simulink model "mcu_flat"  (R2025b)
settings: Solver=FixedStepDiscrete  StartTime=0.0  StopTime=10.0  FixedStep=Ts_inner  RelTol=1e-3
InitFcn:
  | fctrl = init_flatness(quadcop);
  | [mahony, luen] = init_estimator(fctrl.Ts_slow); % Ts_slow = 0.01 = Ts_gcs
  | xi0 = [quadcop.x0; quadcop.v0]; % Luenberger-Startzustand [p;v]
undefined symbols (not defined in the file): imu, luen, mahony, quadcop, safety, supervisor, Ts_batt, Ts_gcs, Ts_inner
settings Model: DataDictionary=project.sldd  Creator=Nick  LastModifiedBy=Rakete
settings SolverCC: AutoInsertRateTranBlk=on
settings OptimizationCC: DefaultParameterBehavior=Inlined  EnhancedBackFolding=on  PassReuseOutputArgsAs=Individual arguments  ZeroExternalMemoryAtStartup=off  ZeroInternalMemoryAtStartup=off  OptimizeBlockOrder=speed  DifferentSizesBufferReuse=on  OptimizationCustomize=off  EfficientTunableParamExpr=on
settings DebuggingCC: ParameterTunabilityLossMsg=error
settings HardwareCC: ProdBitPerPointer=32.0  ProdBitPerSizeT=32.0  ProdBitPerPtrDiffT=32.0  ProdLargestAtomicInteger=Long  ProdLargestAtomicFloat=Double  ProdWordSize=32.0  ProdLongLongMode=on  ProdHWDeviceType=ARM Compatible->ARM Cortex-M
settings SFSimCC: MATLABDynamicMemAlloc=off
settings RTWCC: SystemTargetFile=ert.tlc  GenCodeOnly=on  PackageGeneratedCodeAndArtifacts=on  TemplateMakefile=ert_default_tmf  GenerateReport=on  TargetLang=C++  Description=Embedded Coder
settings CodeAppCC: ForceParamTrailComments=on  IgnoreCustomStorageClasses=off  OperatorAnnotations=on  SimulinkDataObjDesc=on  SFDataObjDesc=on  InsertBlockDesc=on
settings ERTTargetCC: RootIOFormat=Structure reference  ERTCustomFileTemplate=example_file_process.tlc  TargetLangStandard=C++11 (ISO)  GenerateSampleERTMain=on  CodeInterfacePackaging=C++ class  SubcomponentCodeInterfacePackaging=C++ class  SupportNonFinite=off

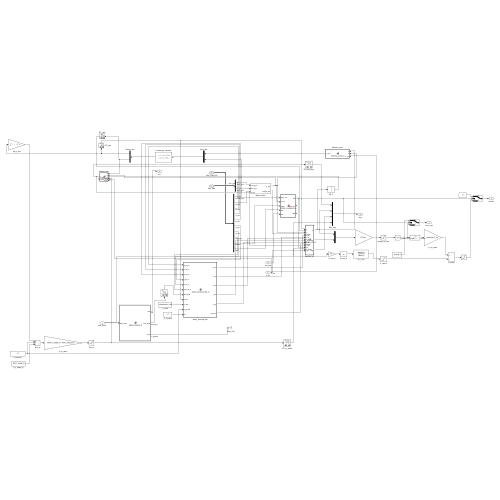
[thumbnail: Simulink's stored preview of the top-level diagram]
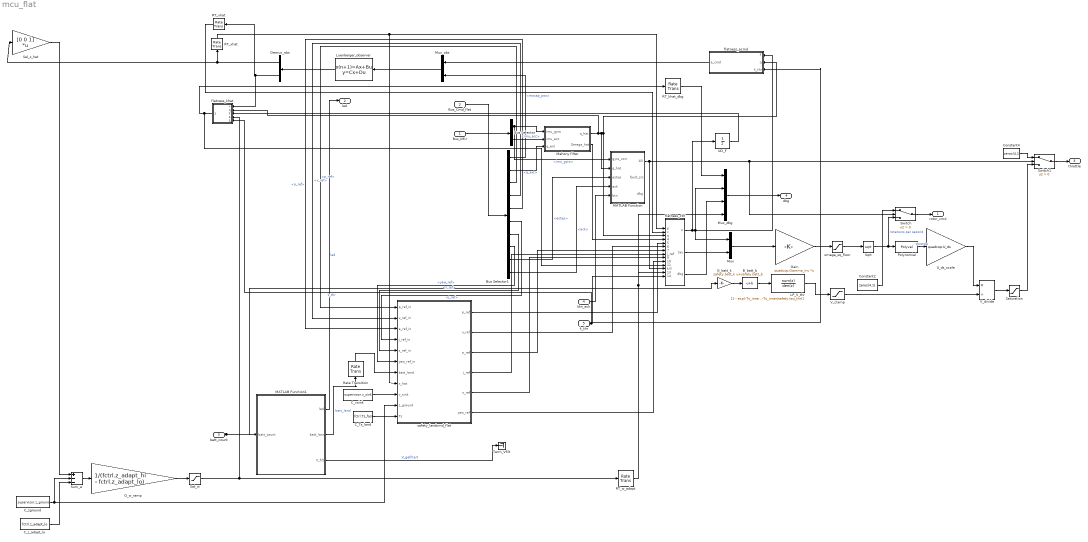
== system mcu_flat ==
  Bus_IMU : Inport  OutDataTypeStr=Bus: Bus_IMU
  Bus_Cmd_flat : Inport  Port=2  OutDataTypeStr=Bus: Bus_Cmd_flat
  batt_count : Inport  Port=3
  btn_ack : Inport  Port=4  OutDataTypeStr=boolean
  k_thr : Inport  Port=5  OutDataTypeStr=double  PortDimensions=1
  B_batt_b : Bias  Bias=safety.batt_b  SaturateOnIntegerOverflow=off
  Bus Selector : BusSelector  OutputSignals=imu_gyro,imu_acc
  Bus Selector1 : BusSelector  OutputSignals=mocap_pos,q_ext,p_ref,v_ref,a_ref,j_ref,s_ref,yaw_ref,estop,ack
  C_Ts_land : Constant  Value=fctrl.Ts_fast
  C_vsink : Constant  Value=supervisor.v_sink
  C_z_adapt_lo : Constant  Value=fctrl.z_adapt_lo
  C_zground : Constant  Value=supervisor.z_ground
  Constant2 : Constant  Value=zeros(4,1)
  Constant4 : Constant  Value=zeros(4,1)
  Demux_obs : Demux  Outputs=2
  G_batt_k : Gain  Gain=safety.batt_k
  G_w_ramp : Gain  Gain=1/(fctrl.z_adapt_hi - fctrl.z_adapt_lo)
  Gain : Gain  Gain=quadcop.Gamma_inv  Multiplication=Matrix(K*u) (u vector)
  LP_V_thr : DiscreteTransferFcn  Numerator=[1 - exp(-Ts_inner/safety.tau_thr)]  Denominator=[1, -exp(-Ts_inner/safety.tau_thr)]  InitialStates=quadcop.V_thr_init  SampleTime=Ts_inner
  Luenberger_observer : DiscreteStateSpace  A=luen.Ad  B=luen.Bd  C=luen.Cd  D=luen.Dd  InitialCondition=xi0  SampleTime=Ts_gcs
  MATLAB Function : MATLAB Function  TreatAsAtomicUnit=on
  MATLAB Function1 : MATLAB Function  TreatAsAtomicUnit=on  SystemSampleTime=Ts_batt
  Mahony filter : Subsystem
  Mux : Mux  Inputs=2
  Mux_dbg : Mux
  Mux_obs : Mux  Inputs=2
  Polynomial : Polyval  Coefs=quadcop.p_from_omega
  RT_khat_dbg : RateTransition  InitialCondition=fctrl.k_hat0
  RT_vhat : RateTransition  OutPortSampleTime=fctrl.Ts_fast
  RT_w_adapt : RateTransition
  RT_xhat : RateTransition  OutPortSampleTime=fctrl.Ts_fast
  Rate Transition : RateTransition  OutPortSampleTime=Ts_inner
  Sat_w : Saturate  UpperLimit=1  LowerLimit=0
  Saturation : Saturate  UpperLimit=100  LowerLimit=0
  Sel_z_hat : Gain  Gain=[0 0 1]  Multiplication=Matrix(K*u)
  Sqrt : Sqrt
  Sum_w : Sum  Inputs=+--
  Switch : Switch  Criteria=u2 > Threshold  SaturateOnIntegerOverflow=off  InputSameDT=off
  Switch1 : Switch  Criteria=u2 > Threshold  SaturateOnIntegerOverflow=off  InputSameDT=off
  Term_Vfilt : Terminator
  UD_F : UnitDelay  InitialCondition=fctrl.m*fctrl.g  SampleTime=fctrl.Ts_fast  HasFrameUpgradeWarning=on
  U_ds_scale : Gain  Gain=quadcop.U_ds
  V_clamp : Saturate  UpperLimit=quadcop.V_thr_max  LowerLimit=quadcop.V_thr_min
  V_divide : Product  Inputs=*/
  flatness_acmd : MATLAB Function  TreatAsAtomicUnit=on
  flatness_ctrl : MATLAB Function  TreatAsAtomicUnit=on  SystemSampleTime=fctrl.Ts_fast
  flatness_khat : MATLAB Function  TreatAsAtomicUnit=on  SystemSampleTime=fctrl.Ts_slow
  omega_sq_floor : Saturate  UpperLimit=inf  LowerLimit=0
  safety_landcmd_flat : MATLAB Function  TreatAsAtomicUnit=on  SystemSampleTime=Ts_inner
  rotor_cmd : Outport
  led : Outport  Port=2
  throttle : Outport  Port=3
  dbg : Outport  Port=4
  wires:
  Bus Selector/1 -> MATLAB Function/1(gyro_corr), Mahony filter/1(imu_gyro)  "<imu_gyro>"
  G_w_ramp/1 -> Sat_w/1
  Constant4/1 -> Switch1/1
  Sum_w/1 -> G_w_ramp/1
  C_z_adapt_lo/1 -> Sum_w/3
  Sel_z_hat/1 -> Sum_w/1
  flatness_khat/1(k_hat) -> flatness_ctrl/11(k_hat), RT_khat_dbg/1
  C_Ts_land/1 -> safety_landcmd_flat/11(Ts)
  C_zground/1 -> safety_landcmd_flat/10(z_ground), Sum_w/2
  Sat_w/1 -> flatness_khat/4(w_adapt), RT_w_adapt/1
  RT_vhat/1 -> flatness_ctrl/2(v)
  Mux_obs/1 -> Luenberger_observer/1
  RT_xhat/1 -> flatness_ctrl/1(p), safety_landcmd_flat/8(x_hat)
  batt_count/1 -> MATLAB Function1/1(batt_count), G_batt_k/1
  Demux_obs/2 -> RT_vhat/1, flatness_khat/1(v)
  Gain/1 -> omega_sq_floor/1
  Demux_obs/1 -> RT_xhat/1, Sel_z_hat/1
  MATLAB Function1/1(led) -> led/1  "led"
  C_vsink/1 -> safety_landcmd_flat/9(v_sink)
  MATLAB Function1/2(batt_land) -> Rate Transition/1  "batt_land"
  omega_sq_floor/1 -> Sqrt/1
  Mux/1 -> Gain/1
  safety_landcmd_flat/6(yaw_ref) -> flatness_ctrl/10(yawref)
  Bus Selector/2 -> Mahony filter/2(imu_acc)  "<imu_acc>"
  Luenberger_observer/1 -> Demux_obs/1
  Constant2/1 -> Switch/1
  safety_landcmd_flat/2(v_ref) -> flatness_ctrl/6(v_ref)
  Rate Transition/1 -> safety_landcmd_flat/7(batt_land)
  Bus_IMU/1 -> Bus Selector/1
  Bus_Cmd_flat/1 -> Bus Selector1/1
  Bus Selector1/5 -> safety_landcmd_flat/3(a_ref_in)  "<a_ref>"
  safety_landcmd_flat/1(p_ref) -> flatness_ctrl/5(p_ref)
  RT_khat_dbg/1 -> Mux_dbg/1
  safety_landcmd_flat/3(a_ref) -> flatness_ctrl/7(a_ref)
  U_ds_scale/1 -> V_divide/1
  Polynomial/1 -> U_ds_scale/1  "throttle"
  Sqrt/1 -> Polynomial/1, Switch/3  "rotations per second"
  Mahony filter/2(Omega_hat) -> flatness_ctrl/4(omega)
  safety_landcmd_flat/4(j_ref) -> flatness_ctrl/8(j_ref)
  btn_ack/1 -> MATLAB Function/5(btn)
  safety_landcmd_flat/5(s_ref) -> flatness_ctrl/9(s_ref)
  Bus Selector1/1 -> Mux_obs/2  "<mocap_pos>"
  V_clamp/1 -> V_divide/2
  Bus Selector1/2 -> Mahony filter/3(q_ext)  "<q_ext>"
  V_divide/1 -> Saturation/1
  Bus Selector1/3 -> safety_landcmd_flat/1(p_ref_in)  "<p_ref>"
  Bus Selector1/4 -> safety_landcmd_flat/2(v_ref_in)  "<v_ref>"
  Bus Selector1/6 -> safety_landcmd_flat/4(j_ref_in)  "<j_ref>"
  RT_w_adapt/1 -> Mux_dbg/4, flatness_ctrl/13(w_adapt)
  Bus Selector1/10 -> MATLAB Function/4(ack)  "<ack>"
  Bus Selector1/7 -> safety_landcmd_flat/5(s_ref_in)  "<s_ref>"
  Bus Selector1/8 -> safety_landcmd_flat/6(yaw_ref_in)  "<yaw_ref>"
  Bus Selector1/9 -> MATLAB Function/3(estop)  "<estop>"
  flatness_ctrl/2(tau) -> Mux/2
  Saturation/1 -> Switch1/3
  UD_F/1 -> flatness_khat/3(F)
  Switch/1 -> rotor_cmd/1
  Mahony filter/1(q_hat) -> flatness_ctrl/3(q), flatness_acmd/2(q), MATLAB Function/2(q_hat), flatness_khat/2(q)
  MATLAB Function/1(kill) -> Switch/2, Switch1/2, flatness_ctrl/12(kill)
  flatness_ctrl/1(F) -> flatness_acmd/1(F), Mux/1, Mux_dbg/2, UD_F/1
  flatness_ctrl/3(dbg) -> Mux_dbg/3
  flatness_acmd/1(a_cmd) -> Mux_obs/1
  Mux_dbg/1 -> dbg/1
  Switch1/1 -> throttle/1
  MATLAB Function1/3(V_filt) -> Term_Vfilt/1  "V_gefiltert"
  G_batt_k/1 -> B_batt_b/1
  B_batt_b/1 -> LP_V_thr/1
  LP_V_thr/1 -> V_clamp/1
  k_thr/1 -> flatness_ctrl/14(k_thr), flatness_khat/5(k_thr), flatness_acmd/3(k_thr)  "k_thr"

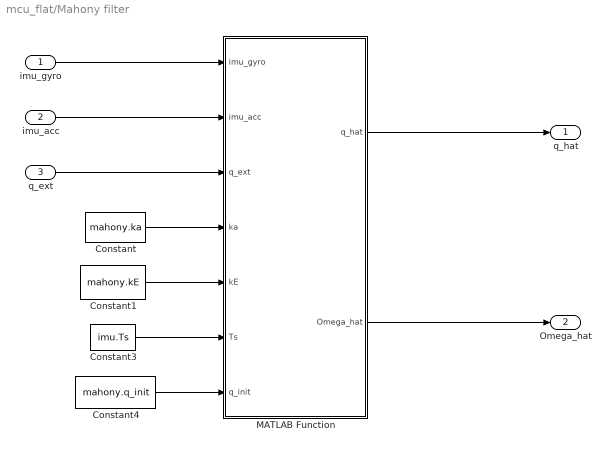
== system mcu_flat/Mahony filter ==
  imu_gyro : Inport
  imu_acc : Inport  Port=2
  q_ext : Inport  Port=3
  Constant : Constant  Value=mahony.ka
  Constant1 : Constant  Value=mahony.kE
  Constant3 : Constant  Value=imu.Ts
  Constant4 : Constant  Value=mahony.q_init
  MATLAB Function : MATLAB Function  TreatAsAtomicUnit=on
  q_hat : Outport
  Omega_hat : Outport  Port=2
  wires:
  MATLAB Function/1(q_hat) -> q_hat/1
  MATLAB Function/2(Omega_hat) -> Omega_hat/1
  imu_gyro/1 -> MATLAB Function/1(imu_gyro)
  imu_acc/1 -> MATLAB Function/2(imu_acc)
  q_ext/1 -> MATLAB Function/3(q_ext)
  Constant/1 -> MATLAB Function/4(ka)
  Constant1/1 -> MATLAB Function/5(kE)
  Constant3/1 -> MATLAB Function/6(Ts)
  Constant4/1 -> MATLAB Function/7(q_init)

== matlab function mcu_flat/safety_landcmd_flat ==
  data: p_ref output; v_ref output; p_ref_in input; a_ref output; j_ref output; v_ref_in input; a_ref_in input; j_ref_in input; s_ref_in input; yaw_ref_in input; batt_land input; s_ref output; x_hat input; v_sink input; z_ground input; Ts input; yaw_ref output
function [p_ref, v_ref, a_ref, j_ref, s_ref, yaw_ref] = safety_landcmd_flat_sl(p_ref_in, v_ref_in, a_ref_in, j_ref_in, s_ref_in, yaw_ref_in, batt_land, x_hat, v_sink, z_ground, Ts)
%#codegen
% WRAPPER — code liegt in
% scripts\flatness\safety_landcmd_flat.m - dieser Block ruft sie nur auf
[p_ref, v_ref, a_ref, j_ref, s_ref, yaw_ref] = safety_landcmd_flat(p_ref_in, v_ref_in, a_ref_in, j_ref_in, s_ref_in, yaw_ref_in, batt_land, x_hat, v_sink, z_ground, Ts);
end

== matlab function mcu_flat/flatness_acmd ==
  data: F input; q input; k_thr input; a_cmd output; fctrl parameter
function a_cmd = flatness_acmd_sl(F, q, k_thr, fctrl)
%#codegen
% WRAPPER — code liegt in
% scripts\flatness\flatness_acmd.m - dieser Block ruft sie nur auf
% k_thr: Schubfaktor je Drohne
a_cmd = flatness_acmd(k_thr*F, q, fctrl.m, fctrl.g);
end

== matlab function mcu_flat/flatness_ctrl ==
  data: p input double size=[3 1]; v input double size=[3 1]; F output double size=[1 1]; q input double size=[4 1]; omega input double size=[3 1]; p_ref input double size=[3 1]; v_ref input double size=[3 1]; a_ref input double size=[3 1]; j_ref input double size=[3 1]; s_ref input double size=[3 1]; yawref input double size=[3 1]; k_hat input double size=[1 1]; kill input; w_adapt input; k_thr input; tau output double size=[3 1]; fctrl parameter; dbg output
function [F, tau, dbg] = flatness_ctrl_sl(p, v, q, omega, p_ref, v_ref, a_ref, j_ref, s_ref, yawref, k_hat, kill, w_adapt, k_thr, fctrl)
%#codegen
% WRAPPER - code liegt in
% scripts\flatness\flatness_ctrl.m - dieser Block ruft sie nur auf
% k_thr: Schubfaktor je Drohne
    [F, tau, dbg] = flatness_ctrl(p, v, q, omega, p_ref, v_ref, a_ref, j_ref, s_ref, yawref, k_hat/k_thr, fctrl.m/k_thr, fctrl.g, fctrl.J, fctrl.coefPos, fctrl.coefPhi, fctrl.Ts_fast, kill, w_adapt);
end

== matlab function mcu_flat/Mahony filter/MATLAB Function ==
  data: imu_gyro input; q_hat output; imu_acc input; q_ext input; ka input; kE input; Ts input; Omega_hat output; q_init input
function [q_hat, Omega_hat] = mahony_filter_sl(imu_gyro, imu_acc, q_ext, ka, kE, Ts, q_init)
%#codegen
% WRAPPER — code liegt in
% scripts\functions\mahony_filter.m - dieser Block ruft sie nur auf
[q_hat, Omega_hat] = mahony_filter(imu_gyro, imu_acc, q_ext, ka, kE, Ts, q_init);
end

== matlab function mcu_flat/MATLAB Function ==
  data: gyro_corr input double size=[3 1]; q_hat input; estop input uint8 size=1; kill output boolean size=1; ack input boolean size=1; btn input; fault_src output uint8 size=1; dbg output size=[3 1]; safety parameter
function [kill, fault_src, dbg] = safety_overspeed_sl(gyro_corr, q_hat, estop, ack, btn, safety)
%#codegen
% WRAPPER  code liegt in
% scripts\functions\safety_overspeed.m - dieser Block ruft sie nur auf
[kill, fault_src, dbg] = safety_overspeed(gyro_corr, q_hat, estop, ack, btn, safety);
end

== matlab function mcu_flat/MATLAB Function1 ==
  data: batt_count input; led output; batt_land output boolean size=[1 1]; V_filt output double size=[1 1]; safety parameter
function [led, batt_land, V_filt] = safety_battery_sl(batt_count, safety)
%#codegen
% WRAPPER — code liegt in
% scripts\functions\safety_battery.m - dieser Block ruft sie nur auf
[led, batt_land, V_filt] = safety_battery(batt_count, safety);
end

== matlab function mcu_flat/flatness_khat ==
  data: v input double size=[3 1]; k_hat output double size=[1 1]; q input double size=[4 1]; F input double size=[1 1]; w_adapt input; k_thr input; fctrl parameter
function k_hat = flatness_khat_sl(v, q, F, w_adapt, k_thr, fctrl)
%#codegen
% WRAPPER - code liegt in
% scripts\flatness\flatness_khat.m - dieser Block ruft sie nur auf
% k_thr: Schubfaktor je Drohne = Startwert
k_hat = flatness_khat(v, q, F, fctrl.m, fctrl.g, fctrl.gamma_khat, fctrl.tau_lp, fctrl.Ts_slow, k_thr, w_adapt);
end
